simulink model "WobblingMassModel"  (R2020b)
settings: Solver=VariableStepAuto  StartTime=0.0  StopTime=5  MaxStep=1e-3  RelTol=1e-3
undefined symbols (not defined in the file or in its folder): p
libraries: simulink x1
settings Model: Creator=Christian Rode  LastModifiedBy=annikaklotz

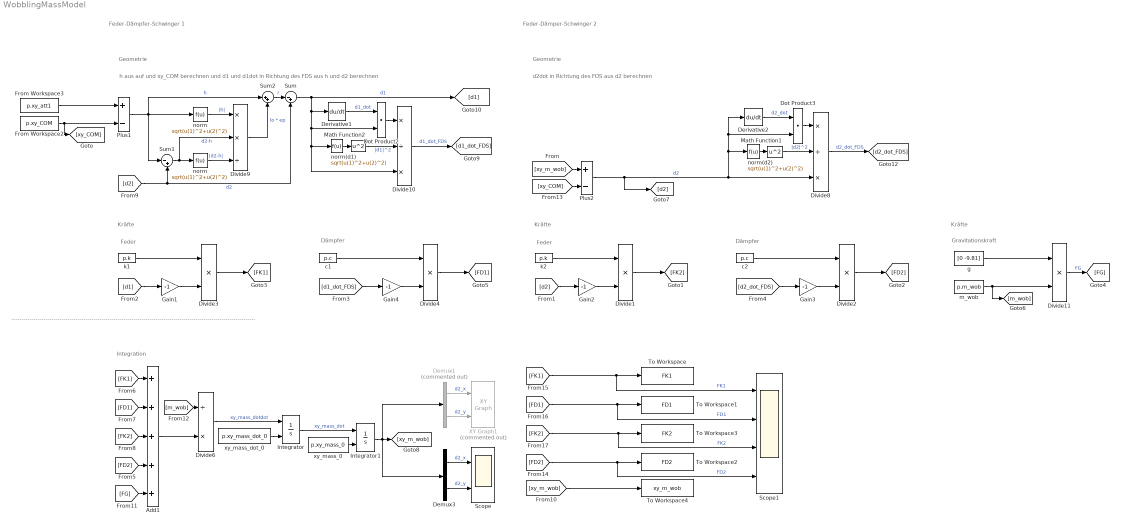
== system WobblingMassModel ==
  note: --------------------------------------------------------------------------------------------------------------------------
  note: h aus auf und xy_COM berechnen und d1 und d1dot in Richtung des FDS aus h und d2 berechnen
  note: Integration
  note: Feder-Dämpfer-Schwinger 1
  note: d2dot in Richtung des FDS aus d2 berechnen
  note: Feder-Dämper-Schwinger 2
  note: Geometrie
  note: Geometrie
  note: Gravitationskraft
  note: Kräfte
  note: Kräfte
  note: Dämpfer
  note: Feder
  note: Kräfte
  note: Dämpfer
  note: Feder
  Add1 : Sum  Inputs=+++++
  Demux1 : Demux  Commented=on  Outputs=2
  Demux3 : Demux  Outputs=2
  Derivative1 : Derivative
  Derivative2 : Derivative
  Divide{1..4,11} (5 alike) : Product  Inputs=**
  Divide10 : Product  Inputs=*/*
  Divide6 : Product  Inputs=/*
  Divide8 : Product  Inputs=*/*
  Divide9 : Product  Inputs=**/
  Dot Product2 : DotProduct  InputSameDT=on  OutDataTypeStr=Inherit: Inherit via internal rule
  Dot Product3 : DotProduct  InputSameDT=on  OutDataTypeStr=Inherit: Inherit via internal rule
  From Workspace2 : FromWorkspace  VariableName=p.xy_COM
  From Workspace3 : FromWorkspace  VariableName=p.xy_att1
  Gain{1..4} (4 alike) : Gain  Gain=-1
  Integrator : Integrator  InitialConditionSource=external
  Integrator1 : Integrator  InitialConditionSource=external
  Math Function1 : Math  Operator=square  SaturateOnIntegerOverflow=on
  Math Function2 : Math  Operator=square  SaturateOnIntegerOverflow=on
  Plus1 : Sum  Inputs=+-
  Plus2 : Sum  Inputs=+-
  Scope : Scope  NumInputPorts=2
  Scope1 : Scope  NumInputPorts=4
  Sum : Sum  Inputs=|-+
  Sum1 : Sum  Inputs=|-+
  Sum2 : Sum  Inputs=|++
  To Workspace : ToWorkspace  VariableName=FK1  SampleTime=-1
  To Workspace1 : ToWorkspace  VariableName=FD1  SampleTime=-1
  To Workspace2 : ToWorkspace  VariableName=FD2  SampleTime=-1
  To Workspace3 : ToWorkspace  VariableName=FK2  SampleTime=-1
  To Workspace4 : ToWorkspace  VariableName=xy_m_wob  SampleTime=-1
  XY Graph1 : simulink/Sinks/XY Graph  Commented=on  xmin=-.2  xmax=.2  ymin=-.2  ymax=.2  st=-1
  c1 : Constant  Value=p.c
  c2 : Constant  Value=p.c
  g : Constant  Value=[0 -9.81]
  k1 : Constant  Value=p.k
  k2 : Constant  Value=p.k
  "m_wob " : Constant  Value=p.m_wob
  norm : Fcn  Expr=sqrt(u(1)^2+u(2)^2)
  "norm " : Fcn  Expr=sqrt(u(1)^2+u(2)^2)
  norm(d1) : Fcn  Expr=sqrt(u(1)^2+u(2)^2)
  norm(d2) : Fcn  Expr=sqrt(u(1)^2+u(2)^2)
  xy_mass_0 : Constant  Value=p.xy_mass_0
  xy_mass_dot_0 : Constant  Value=p.xy_mass_dot_0
  wires:
  Integrator/1 -> Integrator1/1  "xy_mass_dot"
  xy_mass_dot_0/1 -> Integrator/2
  [FK1] -> Add1/1
  [FD1] -> Add1/2
  [FK2] -> Add1/3
  Add1/1 -> Divide6/2
  Divide6/1 -> Integrator/1  "xy_mass_dotdot"
  Demux1/1 -> XY Graph1/1  "d2_x"
  Demux1/2 -> XY Graph1/2  "d2_y"
  "norm "/1 -> Divide9/3  "|d2-h|"
  Divide9/1 -> Sum2/2  "lo * ep"
  [d2] -> Sum/2, Sum1/2  "d2"
  norm/1 -> Divide9/1  "|h|"
  Sum1/1 -> "norm "/1, Divide9/2  "d2-h"
  Sum2/1 -> Sum/1  "r"
  Math Function2/1 -> Divide10/2  "|d1|^2"
  Dot Product2/1 -> Divide10/1
  Divide10/1 -> [d1_dot_FDS]  "d1_dot_FDS"
  norm(d1)/1 -> Math Function2/1
  Derivative1/1 -> Dot Product2/1  "d1_dot"
  Sum/1 -> Divide10/3, norm(d1)/1, Dot Product2/2, Derivative1/1, [d1]  "d1"
  Plus2/1 -> [d2], Derivative2/1, Dot Product3/2, norm(d2)/1, Divide8/3  "d2"
  Math Function1/1 -> Divide8/2  "|d2|^2"
  Dot Product3/1 -> Divide8/1
  norm(d2)/1 -> Math Function1/1
  Derivative2/1 -> Dot Product3/1  "d2_dot"
  Divide8/1 -> [d2_dot_FDS]  "d2_dot_FDS"
  Divide11/1 -> [FG]  "FG"
  g/1 -> Divide11/1
  [d1_dot_FDS] -> Gain4/1
  c1/1 -> Divide4/1
  Gain4/1 -> Divide4/2
  Divide4/1 -> [FD1]
  Gain1/1 -> Divide3/2
  [d1] -> Gain1/1
  Divide3/1 -> [FK1]
  k1/1 -> Divide3/1
  Gain3/1 -> Divide2/2
  Divide2/1 -> [FD2]
  k2/1 -> Divide1/1
  c2/1 -> Divide2/1
  [d2_dot_FDS] -> Gain3/1
  Gain2/1 -> Divide1/2
  [d2] -> Gain2/1
  Divide1/1 -> [FK2]
  [FD2] -> Add1/4
  [FG] -> Add1/5
  [m_wob] -> Divide6/1
  Integrator1/1 -> Demux1/1, Demux3/1, [xy_m_wob]
  Demux3/1 -> Scope/1  "d2_x"
  Demux3/2 -> Scope/2  "d2_y"
  [FK1] -> Scope1/1, To Workspace/1  "FK1"
  [FD1] -> To Workspace1/1, Scope1/2  "FD1"
  [FK2] -> To Workspace3/1, Scope1/3  "FK2"
  [FD2] -> To Workspace2/1, Scope1/4  "FD2"
  Plus1/1 -> Sum2/1, Sum1/1, norm/1  "h"
  From Workspace3/1 -> Plus1/1
  From Workspace2/1 -> [xy_COM], Plus1/2
  xy_mass_0/1 -> Integrator1/2
  [xy_m_wob] -> Plus2/1
  [xy_COM] -> Plus2/2
  "m_wob "/1 -> [m_wob], Divide11/2
  [xy_m_wob] -> To Workspace4/1
